simulink model "sum4"  (Simulink 7.4)
settings: Solver=ode45  StartTime=0.0  StopTime=10.0  RelTol=1e-3
settings Model: Creator=autologin  LastModifiedBy=autologin

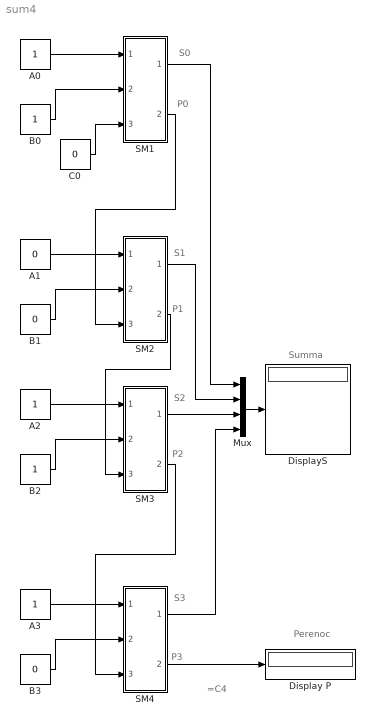
== system sum4 ==
  note: Summa
  note: Perenoc
  note: S0
  note: P0
  note: S1
  note: S2
  note: S3
  note: P1
  note: P2
  note: P3
  note: =C4
  A0 : Constant  OutDataType=fixdt(1, 16)  OutScaling=2^0
  A1 : Constant  Value=0  OutDataType=fixdt(1, 16)  OutScaling=2^0
  A2 : Constant  OutDataType=fixdt(1, 16)  OutScaling=2^0
  A3 : Constant  OutDataType=fixdt(1, 16)  OutScaling=2^0
  B0 : Constant  OutDataType=fixdt(1, 16)  OutScaling=2^0
  B1 : Constant  Value=0  OutDataType=fixdt(1, 16)  OutScaling=2^0
  B2 : Constant  OutDataType=fixdt(1, 16)  OutScaling=2^0
  B3 : Constant  Value=0  OutDataType=fixdt(1, 16)  OutScaling=2^0
  C0 : Constant  Value=0  OutDataType=fixdt(1, 16)  OutScaling=2^0
  Display P : Display
  DisplayS : Display
  Mux : Mux
  SM1 : Subsystem
  SM2 : Subsystem
  SM3 : Subsystem
  SM4 : Subsystem
  wires:
  A0/1 -> SM1/1(In1)
  B0/1 -> SM1/2(In2)
  C0/1 -> SM1/3(In3)
  A1/1 -> SM2/1(In1)
  B1/1 -> SM2/2(In2)
  A2/1 -> SM3/1(In1)
  B2/1 -> SM3/2(In2)
  SM1/2(Out2) -> SM2/3(In3)
  A3/1 -> SM4/1(In1)
  B3/1 -> SM4/2(In2)
  SM2/2(Out2) -> SM3/3(In3)
  SM3/2(Out2) -> SM4/3(In3)
  SM4/2(Out2) -> Display P/1
  Mux/1 -> DisplayS/1
  SM1/1(Out1) -> Mux/1
  SM2/1(Out1) -> Mux/2
  SM3/1(Out1) -> Mux/3
  SM4/1(Out1) -> Mux/4

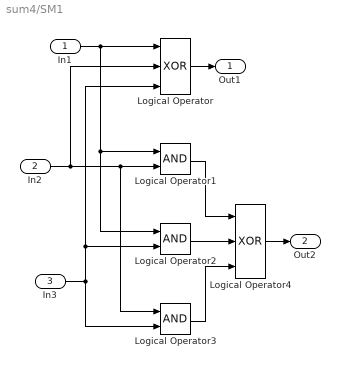
== system sum4/SM1 ==
  In1 : Inport
  In2 : Inport  Port=2
  In3 : Inport  Port=3
  Logical Operator : Logic  Operator=XOR  Inputs=3  AllPortsSameDT=off  OutDataTypeMode=boolean  LogicDataType=fixdt(0, 8)  OutDataTypeStr=boolean
  Logical Operator1 : Logic  AllPortsSameDT=off  OutDataTypeMode=boolean  LogicDataType=fixdt(0, 8)  OutDataTypeStr=boolean
  Logical Operator2 : Logic  AllPortsSameDT=off  OutDataTypeMode=boolean  LogicDataType=fixdt(0, 8)  OutDataTypeStr=boolean
  Logical Operator3 : Logic  AllPortsSameDT=off  OutDataTypeMode=boolean  LogicDataType=fixdt(0, 8)  OutDataTypeStr=boolean
  Logical Operator4 : Logic  Operator=XOR  Inputs=3  AllPortsSameDT=off  OutDataTypeMode=boolean  LogicDataType=fixdt(0, 8)  OutDataTypeStr=boolean
  Out1 : Outport
  Out2 : Outport  Port=2
  wires:
  In1/1 -> Logical Operator2/1, Logical Operator1/1, Logical Operator/1
  In2/1 -> Logical Operator3/1, Logical Operator1/2, Logical Operator/2
  In3/1 -> Logical Operator3/2, Logical Operator2/2, Logical Operator/3
  Logical Operator1/1 -> Logical Operator4/1
  Logical Operator2/1 -> Logical Operator4/2
  Logical Operator3/1 -> Logical Operator4/3
  Logical Operator/1 -> Out1/1
  Logical Operator4/1 -> Out2/1

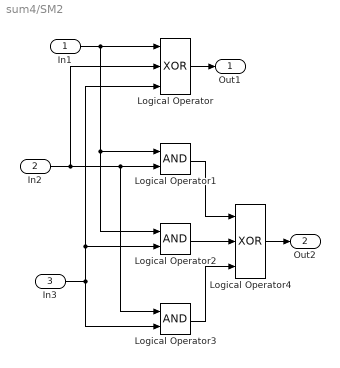
== system sum4/SM2 ==
  In1 : Inport
  In2 : Inport  Port=2
  In3 : Inport  Port=3
  Logical Operator : Logic  Operator=XOR  Inputs=3  AllPortsSameDT=off  OutDataTypeMode=boolean  LogicDataType=fixdt(0, 8)  OutDataTypeStr=boolean
  Logical Operator1 : Logic  AllPortsSameDT=off  OutDataTypeMode=boolean  LogicDataType=fixdt(0, 8)  OutDataTypeStr=boolean
  Logical Operator2 : Logic  AllPortsSameDT=off  OutDataTypeMode=boolean  LogicDataType=fixdt(0, 8)  OutDataTypeStr=boolean
  Logical Operator3 : Logic  AllPortsSameDT=off  OutDataTypeMode=boolean  LogicDataType=fixdt(0, 8)  OutDataTypeStr=boolean
  Logical Operator4 : Logic  Operator=XOR  Inputs=3  AllPortsSameDT=off  OutDataTypeMode=boolean  LogicDataType=fixdt(0, 8)  OutDataTypeStr=boolean
  Out1 : Outport
  Out2 : Outport  Port=2
  wires:
  In1/1 -> Logical Operator2/1, Logical Operator1/1, Logical Operator/1
  In2/1 -> Logical Operator3/1, Logical Operator1/2, Logical Operator/2
  In3/1 -> Logical Operator3/2, Logical Operator2/2, Logical Operator/3
  Logical Operator1/1 -> Logical Operator4/1
  Logical Operator2/1 -> Logical Operator4/2
  Logical Operator3/1 -> Logical Operator4/3
  Logical Operator/1 -> Out1/1
  Logical Operator4/1 -> Out2/1

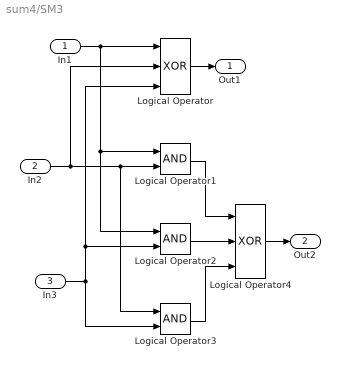
== system sum4/SM3 ==
  In1 : Inport
  In2 : Inport  Port=2
  In3 : Inport  Port=3
  Logical Operator : Logic  Operator=XOR  Inputs=3  AllPortsSameDT=off  OutDataTypeMode=boolean  LogicDataType=fixdt(0, 8)  OutDataTypeStr=boolean
  Logical Operator1 : Logic  AllPortsSameDT=off  OutDataTypeMode=boolean  LogicDataType=fixdt(0, 8)  OutDataTypeStr=boolean
  Logical Operator2 : Logic  AllPortsSameDT=off  OutDataTypeMode=boolean  LogicDataType=fixdt(0, 8)  OutDataTypeStr=boolean
  Logical Operator3 : Logic  AllPortsSameDT=off  OutDataTypeMode=boolean  LogicDataType=fixdt(0, 8)  OutDataTypeStr=boolean
  Logical Operator4 : Logic  Operator=XOR  Inputs=3  AllPortsSameDT=off  OutDataTypeMode=boolean  LogicDataType=fixdt(0, 8)  OutDataTypeStr=boolean
  Out1 : Outport
  Out2 : Outport  Port=2
  wires:
  In1/1 -> Logical Operator2/1, Logical Operator1/1, Logical Operator/1
  In2/1 -> Logical Operator3/1, Logical Operator1/2, Logical Operator/2
  In3/1 -> Logical Operator3/2, Logical Operator2/2, Logical Operator/3
  Logical Operator1/1 -> Logical Operator4/1
  Logical Operator2/1 -> Logical Operator4/2
  Logical Operator3/1 -> Logical Operator4/3
  Logical Operator/1 -> Out1/1
  Logical Operator4/1 -> Out2/1

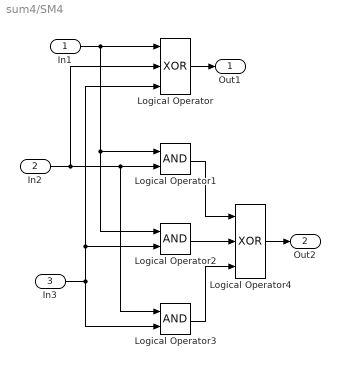
== system sum4/SM4 ==
  In1 : Inport
  In2 : Inport  Port=2
  In3 : Inport  Port=3
  Logical Operator : Logic  Operator=XOR  Inputs=3  AllPortsSameDT=off  OutDataTypeMode=boolean  LogicDataType=fixdt(0, 8)  OutDataTypeStr=boolean
  Logical Operator1 : Logic  AllPortsSameDT=off  OutDataTypeMode=boolean  LogicDataType=fixdt(0, 8)  OutDataTypeStr=boolean
  Logical Operator2 : Logic  AllPortsSameDT=off  OutDataTypeMode=boolean  LogicDataType=fixdt(0, 8)  OutDataTypeStr=boolean
  Logical Operator3 : Logic  AllPortsSameDT=off  OutDataTypeMode=boolean  LogicDataType=fixdt(0, 8)  OutDataTypeStr=boolean
  Logical Operator4 : Logic  Operator=XOR  Inputs=3  AllPortsSameDT=off  OutDataTypeMode=boolean  LogicDataType=fixdt(0, 8)  OutDataTypeStr=boolean
  Out1 : Outport
  Out2 : Outport  Port=2
  wires:
  In1/1 -> Logical Operator2/1, Logical Operator1/1, Logical Operator/1
  In2/1 -> Logical Operator3/1, Logical Operator1/2, Logical Operator/2
  In3/1 -> Logical Operator3/2, Logical Operator2/2, Logical Operator/3
  Logical Operator1/1 -> Logical Operator4/1
  Logical Operator2/1 -> Logical Operator4/2
  Logical Operator3/1 -> Logical Operator4/3
  Logical Operator/1 -> Out1/1
  Logical Operator4/1 -> Out2/1
